simulink library "DSCdq_Library"  (R2018a)
settings: Solver=VariableStepAuto  StartTime=0.0  StopTime=10.0  RelTol=1e-3
values from neighbouring files (symbols this model uses):
  Ts = Ts_control / 60    (= 9.25925925926e-07)    [Equivalency_Script.m]    (also in FreqAdaptiveFFT_Script.m; FreqAdaptive_Script.m; ShortPulse_Script.m)
undefined symbols (not defined in the file or in its folder): ESS, PCC
libraries: $bdroot x20, powerlib_meascontrol x16, powerlib x3, cstblocks x2
settings Model: Creator=daniemot  LastModifiedBy=daniemot

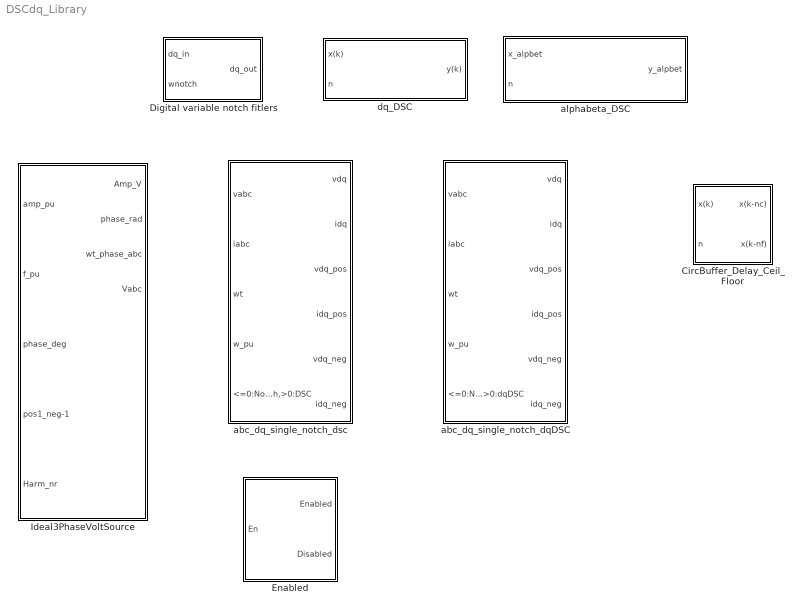
== system DSCdq_Library ==
  CircBuffer_Delay_Ceil_Floor : Subsystem  TreatAsAtomicUnit=on  SystemSampleTime=Ts  mask(Circular buffer with two variable delays (ceiling and floor)){Ts=Ts, nmax=200}
      mask prompts: Ts "Sampling time [s]"; nmax "Circular buffer length"
      mask help:
      | Circular Buffer
      | By: Mota
      | Revision history:	2021-07-16: first release
      |
      | Interface
      | Inputs
      | 	x : must be a vector pf two values
      | 	n : delay in samples (float, ideal delay is time was continuous)
      | 	nmax : max size of circular buffer, ONLY used in FIRST CYCLE
      |
      | Output
      | 	yc = x(k - ceil(n))
      | 	yf = x(k - floor(n))
  Digital variable notch fitlers : Subsystem  mask{Ts=Ts, zeta=0.707}
      mask prompts: Ts "Sampling time [s]"; zeta "Damping factor zeta for notches"
  Enabled : Subsystem  SystemSampleTime=Ts  mask(Enabled block){}
      mask help:
      | if En > 0
      |     Enabled = 1;
      |     Disabled = 0;
      | else
      |     Enabled = 0;
      |     Disabled = 1;
      | end
      mask Display: fprintf('Enable');
  Ideal3PhaseVoltSource : Subsystem  mask(Three-phase ideal voltage source){BaseAmp=1, fn=50}
      mask prompts: BaseAmp "Base phase-to-neutral amplitude [V]"; fn "Base frequency [Hz]"
      mask help:
      | Three-phase balanced ideal voltage source with neutral point not connected.
      |
      | The voltage source can be connected in series with others.
      |
      | va [V] = amp_pu*BaseAmp*sin(2*pi*(f_pu/s)*Harm_nr + Harm_nr*phase_deg*pi/180)
      | vb [V] = ... + Harm_nr*Ph_b_sign*2*pi/3)
      | vc [V] = ... + Harm_nr*Ph_c_sign*2*pi/3)
      |
      | If Pos1_Neg-1 = 1
      | 	Ph_b_sign = -1
      | 	Ph_c_sign = +1
      |
      | If Pos1_Neg-1 = -1
      | 	Ph_b_sign = +1
      | 	Ph_c_sign = -1
  abc_dq_single_notch_dqDSC : Subsystem  mask(abc->dq with Matlab){Ts=0.001, fn=50, fmin=40, zeta=0.707}
      mask prompts: Ts "Sampling time [s]"; fn "Grid frequency [Hz]"; fmin "Min. acceptable grid freq. [Hz]"; zeta "Zeta for notch filters"
      mask help:
      | To be done
      |
      | Max buffer size for DSC 500 samples
  abc_dq_single_notch_dsc : Subsystem  mask(abc->dq with Matlab){Ts=0.001, fn=50, fmin=40, zeta=0.707}
      mask prompts: Ts "Sampling time [s]"; fn "Rated grid frequency [Hz]"; fmin "Min. acceptable grid freq. [Hz]"; zeta "Zeta for notch filters"
      mask help:
      | To be done
      |
      | Max buffer size for DSC 500 samples
  alphabeta_DSC : Subsystem  mask{Ts=Ts, nmax=200}
      mask prompts: Ts "Sample times [s]"; nmax "Maximum delay nmax:"
      mask Display: fprintf('y(k)=0.5(x(k)+jx(k-n))');
  dq_DSC : Subsystem  mask{Ts=Ts, nmax=200}
      mask prompts: Ts "Sample times [s]"; nmax "Maximum delay nmax:"
      mask Display: fprintf('y(k)=0.5(x(k)+x(k-n))');

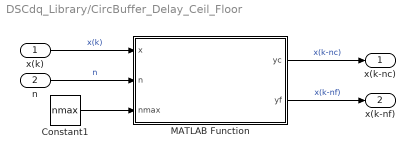
== system DSCdq_Library/CircBuffer_Delay_Ceil_Floor ==
  x(k) : Inport
  n : Inport  Port=2
  Constant1 : Constant  Value=nmax
  MATLAB Function : MATLAB Function  TreatAsAtomicUnit=on  SystemSampleTime=Ts
  x(k-nc) : Outport
  x(k-nf) : Outport  Port=2
  wires:
  n/1 -> MATLAB Function/2(n)  "n"
  MATLAB Function/2(yf) -> x(k-nf)/1  "x(k-nf)"
  x(k)/1 -> MATLAB Function/1(x)  "x(k)"
  MATLAB Function/1(yc) -> x(k-nc)/1  "x(k-nc)"
  Constant1/1 -> MATLAB Function/3(nmax)

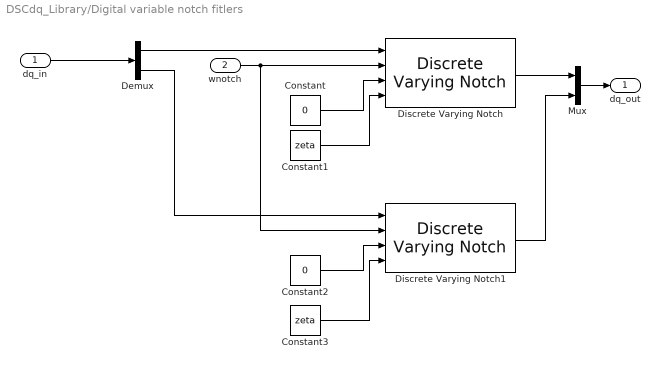
== system DSCdq_Library/Digital variable notch fitlers ==
  dq_in : Inport
  wnotch : Inport  Port=2
  Constant : Constant  Value=0
  Constant1 : Constant  Value=zeta
  Constant2 : Constant  Value=0
  Constant3 : Constant  Value=zeta
  Demux : Demux  Outputs=2
  Discrete Varying Notch : cstblocks/Linear Parameter Varying/Discrete Varying Notch  w0=0  Ts=Ts
      settings: SourceProductName=Control System Toolbox  SourceProductBaseCode=CT
  Discrete Varying Notch1 : cstblocks/Linear Parameter Varying/Discrete Varying Notch  w0=0  Ts=Ts
      settings: SourceProductName=Control System Toolbox  SourceProductBaseCode=CT
  Mux : Mux  Inputs=2
  dq_out : Outport
  wires:
  Constant/1 -> Discrete Varying Notch/3
  Constant1/1 -> Discrete Varying Notch/4
  Demux/2 -> Discrete Varying Notch1/1
  dq_in/1 -> Demux/1
  Constant2/1 -> Discrete Varying Notch1/3
  wnotch/1 -> Discrete Varying Notch1/2, Discrete Varying Notch/2
  Constant3/1 -> Discrete Varying Notch1/4
  Demux/1 -> Discrete Varying Notch/1
  Discrete Varying Notch/1 -> Mux/1
  Mux/1 -> dq_out/1
  Discrete Varying Notch1/1 -> Mux/2

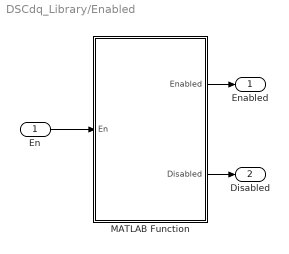
== system DSCdq_Library/Enabled ==
  En : Inport
  MATLAB Function : MATLAB Function  SystemSampleTime=Ts
      settings: RTWSystemCode=Inline
  Enabled : Outport
  Disabled : Outport  Port=2
  wires:
  En/1 -> MATLAB Function/1(En)
  MATLAB Function/1(Enabled) -> Enabled/1
  MATLAB Function/2(Disabled) -> Disabled/1

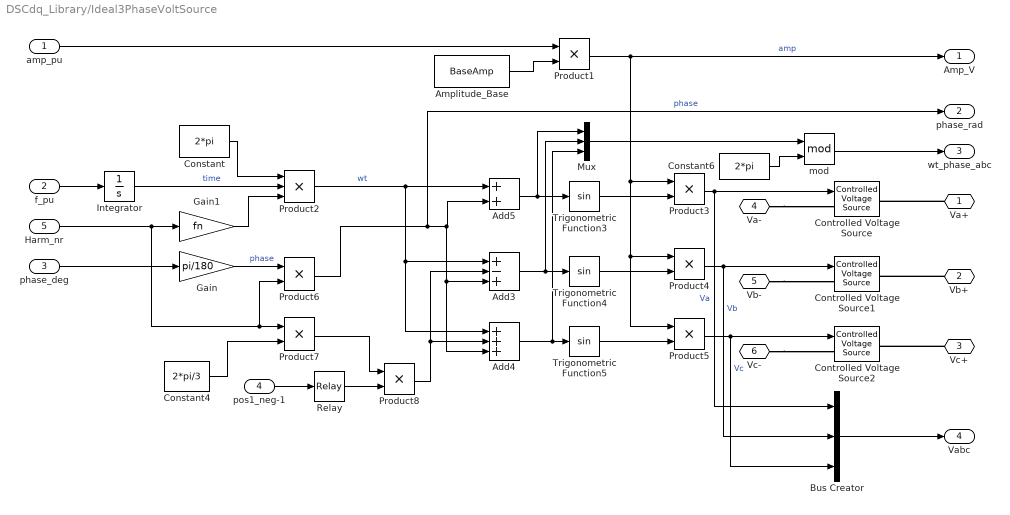
== system DSCdq_Library/Ideal3PhaseVoltSource ==
  amp_pu : Inport
  f_pu : Inport  Port=2
  phase_deg : Inport  Port=3
  pos1_neg-1 : Inport  Port=4
  Harm_nr : Inport  Port=5
  Add3 : Sum  Inputs=+-+
  Add4 : Sum  Inputs=+++
  Add5 : Sum
  Amplitude_Base : Constant  Value=BaseAmp
  Bus Creator : BusCreator  Inputs=3
  Constant : Constant  Value=2*pi
  Constant4 : Constant  Value=2*pi/3
  Constant6 : Constant  Value=2*pi
  Controlled Voltage Source : powerlib/Electrical Sources/Controlled Voltage Source  Initialize=off  Source_Type=AC  Amplitude=ESS.LSC.Ub*(2/3)^0.5  Phase=0  Frequency=PCC.fn  Measurements=None
  Controlled Voltage Source1 : powerlib/Electrical Sources/Controlled Voltage Source  Initialize=off  Source_Type=AC  Amplitude=ESS.LSC.Ub*(2/3)^0.5  Phase=-120  Frequency=PCC.fn  Measurements=None
  Controlled Voltage Source2 : powerlib/Electrical Sources/Controlled Voltage Source  Initialize=off  Source_Type=AC  Amplitude=ESS.LSC.Ub*(2/3)^0.5  Phase=120  Frequency=PCC.fn  Measurements=None
  Gain : Gain  Gain=pi/180
  Gain1 : Gain  Gain=fn
  Integrator : Integrator
  Mux : Mux  Inputs=3
  Product{1,3..8} (7 alike) : Product
  Product2 : Product  Inputs=3
  Relay : Relay  OnSwitchValue=0  OffSwitchValue=-0.1  OffOutputValue=-1
  Trigonometric Function3 : Trigonometry
  Trigonometric Function4 : Trigonometry
  Trigonometric Function5 : Trigonometry
  mod : Math  Operator=mod  SaturateOnIntegerOverflow=on
  Va+ : PMIOPort  Side=Right
  Vb+ : PMIOPort  Port=2  Side=Right
  Vc+ : PMIOPort  Port=3  Side=Right
  Va- : PMIOPort  Port=4  Side=Right
  Vb- : PMIOPort  Port=5  Side=Right
  Vc- : PMIOPort  Port=6  Side=Right
  Amp_V : Outport
  phase_rad : Outport  Port=2
  wt_phase_abc : Outport  Port=3
  Vabc : Outport  Port=4
  wires:
  Add4/1 -> Mux/3, Trigonometric Function5/1
  Product6/1 -> phase_rad/1, Add4/3, Add3/3, Add5/2  "phase"
  Add3/1 -> Mux/2, Trigonometric Function4/1
  pos1_neg-1/1 -> Relay/1
  Product3/1 -> Bus Creator/1, Controlled Voltage Source/1  "Va"
  amp_pu/1 -> Product1/1
  Product8/1 -> Add3/2, Add4/2
  Product5/1 -> Bus Creator/3, Controlled Voltage Source2/1  "Vc"
  Product4/1 -> Bus Creator/2, Controlled Voltage Source1/1  "Vb"
  Amplitude_Base/1 -> Product1/2
  Product7/1 -> Product8/1
  Product1/1 -> Product5/1, Product4/1, Product3/1, Amp_V/1  "amp"
  Relay/1 -> Product8/2
  Trigonometric Function3/1 -> Product3/2
  Product2/1 -> Add5/1, Add4/1, Add3/1  "wt"
  Trigonometric Function5/1 -> Product5/2
  Add5/1 -> Mux/1, Trigonometric Function3/1
  Trigonometric Function4/1 -> Product4/2
  phase_deg/1 -> Gain/1
  f_pu/1 -> Integrator/1
  Constant/1 -> Product2/1
  Gain1/1 -> Product2/3
  Bus Creator/1 -> Vabc/1
  Constant6/1 -> mod/2
  mod/1 -> wt_phase_abc/1
  Gain/1 -> Product6/1  "phase"
  Constant4/1 -> Product7/2
  Mux/1 -> mod/1
  Harm_nr/1 -> Product7/1, Product6/2, Gain1/1
  Integrator/1 -> Product2/2  "time"
  connections:
  Vb+/RConn1 -- Controlled Voltage Source1/RConn1
  Vc+/RConn1 -- Controlled Voltage Source2/RConn1
  Va+/RConn1 -- Controlled Voltage Source/RConn1
  Va-/RConn1 -- Controlled Voltage Source/LConn1
  Vb-/RConn1 -- Controlled Voltage Source1/LConn1
  Vc-/RConn1 -- Controlled Voltage Source2/LConn1

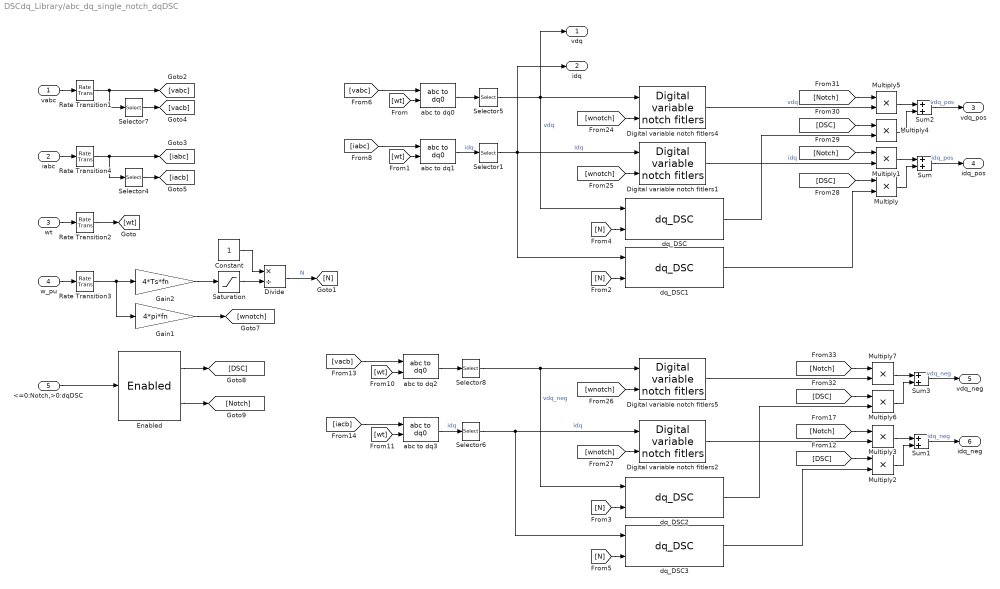
== system DSCdq_Library/abc_dq_single_notch_dqDSC ==
  vabc : Inport
  iabc : Inport  Port=2
  wt : Inport  Port=3
  w_pu : Inport  Port=4
  <=0:Notch,>0:dqDSC : Inport  Port=5
  Constant : Constant
  Digital variable notch fitlers{1..2,4..5} (4 alike) : $bdroot/Digital variable notch fitlers  Ts=Ts  zeta=zeta
  Divide : Product  Inputs=*/
  Enabled : $bdroot/Enabled
  Gain1 : Gain  Gain=4*pi*fn
  Gain2 : Gain  Gain=4*Ts*fn
  Multiply{,1..7} (8 alike) : Product
  Rate Transition1 : RateTransition  OutPortSampleTime=Ts
  Rate Transition2 : RateTransition  OutPortSampleTime=Ts
  Rate Transition3 : RateTransition  InitialCondition=1  OutPortSampleTime=Ts
  Rate Transition4 : RateTransition  OutPortSampleTime=Ts
  Saturation : Saturate  UpperLimit=inf  LowerLimit=0.000001
  Selector{1,5..6,8} (4 alike) : Selector  InputPortWidth=3  IndexOptions=Index vector (dialog)  Indices=[1 2]  OutputSizes=1
  Selector4 : Selector  InputPortWidth=3  IndexOptions=Index vector (dialog)  Indices=[1 3 2]  OutputSizes=1
  Selector7 : Selector  InputPortWidth=3  IndexOptions=Index vector (dialog)  Indices=[1 3 2]  OutputSizes=1
  Sum{,1..3} (4 alike) : Sum
  abc to dq{0..3} (4 alike) : powerlib_meascontrol/Transformations/abc to dq0  Alignment=90 degrees behind phase A axis
  dq_DSC{,1..3} (4 alike) : $bdroot/dq_DSC  Ts=Ts  nmax=round(1/(4*fmin*Ts))
  vdq : Outport
  idq : Outport  Port=2
  vdq_pos : Outport  Port=3
  idq_pos : Outport  Port=4
  vdq_neg : Outport  Port=5
  idq_neg : Outport  Port=6
  wires:
  wt/1 -> Rate Transition2/1
  abc to dq1/1 -> Selector1/1  "idq"
  Selector5/1 -> Digital variable notch fitlers4/1, vdq/1, dq_DSC/1  "vdq"
  abc to dq0/1 -> Selector5/1
  Selector1/1 -> Digital variable notch fitlers1/1, idq/1, dq_DSC1/1  "idq"
  [vabc] -> abc to dq0/1
  [iabc] -> abc to dq1/1
  vabc/1 -> Rate Transition1/1
  iabc/1 -> Rate Transition4/1
  Digital variable notch fitlers4/1 -> Multiply5/2  "vdq"
  Digital variable notch fitlers1/1 -> Multiply1/2  "idq"
  Sum2/1 -> vdq_pos/1  "vdq_pos"
  Sum/1 -> idq_pos/1  "idq_pos"
  Rate Transition2/1 -> [wt]
  [wt] -> abc to dq0/2
  [wt] -> abc to dq1/2
  Divide/1 -> [N]  "N"
  Rate Transition1/1 -> Selector7/1, [vabc]
  Selector7/1 -> [vacb]
  Rate Transition4/1 -> Selector4/1, [iabc]
  Selector4/1 -> [iacb]
  [wt] -> abc to dq3/2
  abc to dq2/1 -> Selector8/1
  Selector8/1 -> Digital variable notch fitlers5/1, dq_DSC2/1  "vdq_neg"
  [vacb] -> abc to dq2/1
  [wt] -> abc to dq2/2
  abc to dq3/1 -> Selector6/1  "idq"
  [iacb] -> abc to dq3/1
  Sum3/1 -> vdq_neg/1  "vdq_neg"
  Sum1/1 -> idq_neg/1  "idq_neg"
  Digital variable notch fitlers5/1 -> Multiply7/2
  Selector6/1 -> Digital variable notch fitlers2/1, dq_DSC3/1  "idq"
  Digital variable notch fitlers2/1 -> Multiply3/2
  dq_DSC3/1 -> Multiply2/2
  Gain2/1 -> Saturation/1
  Saturation/1 -> Divide/2
  Constant/1 -> Divide/1
  Rate Transition3/1 -> Gain1/1, Gain2/1
  w_pu/1 -> Rate Transition3/1
  Gain1/1 -> [wnotch]
  [wnotch] -> Digital variable notch fitlers4/2
  [wnotch] -> Digital variable notch fitlers1/2
  [wnotch] -> Digital variable notch fitlers5/2
  [wnotch] -> Digital variable notch fitlers2/2
  <=0:Notch,>0:dqDSC/1 -> Enabled/1
  Enabled/1 -> [DSC]
  Enabled/2 -> [Notch]
  [DSC] -> Multiply/1
  [Notch] -> Multiply1/1
  Multiply1/1 -> Sum/1
  Multiply/1 -> Sum/2
  [Notch] -> Multiply3/1
  [DSC] -> Multiply2/1
  Multiply3/1 -> Sum1/1
  Multiply2/1 -> Sum1/2
  [Notch] -> Multiply5/1
  Multiply4/1 -> Sum2/2
  [DSC] -> Multiply4/1
  Multiply5/1 -> Sum2/1
  [Notch] -> Multiply7/1
  Multiply6/1 -> Sum3/2
  [DSC] -> Multiply6/1
  Multiply7/1 -> Sum3/1
  [N] -> dq_DSC/2
  [N] -> dq_DSC1/2
  dq_DSC1/1 -> Multiply/2
  [N] -> dq_DSC3/2
  dq_DSC/1 -> Multiply4/2
  [N] -> dq_DSC2/2
  dq_DSC2/1 -> Multiply6/2

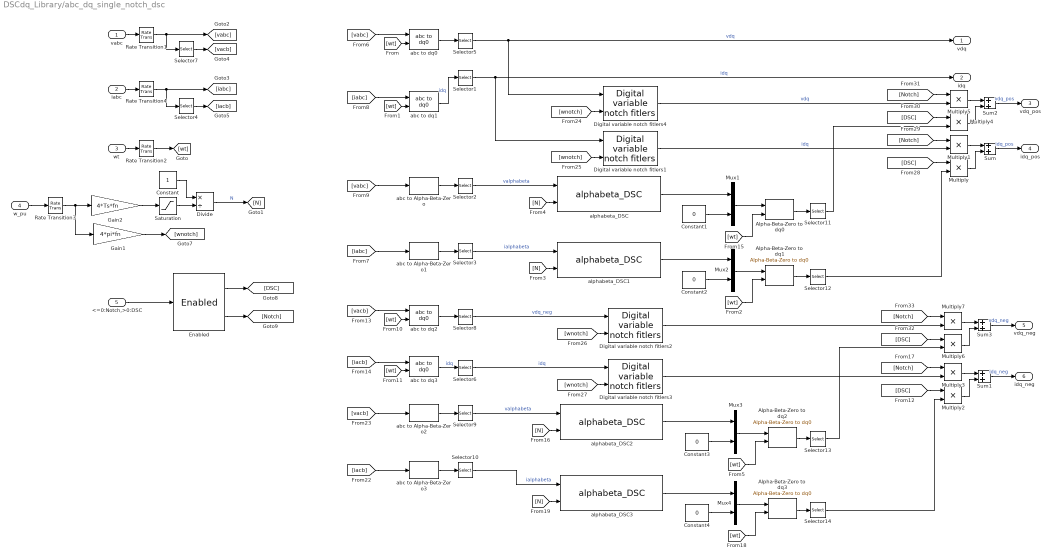
== system DSCdq_Library/abc_dq_single_notch_dsc ==
  vabc : Inport
  iabc : Inport  Port=2
  wt : Inport  Port=3
  w_pu : Inport  Port=4
  <=0:Notch,>0:DSC : Inport  Port=5
  Alpha-Beta-Zero to dq{0..3} (4 alike) : powerlib_meascontrol/Transformations/Alpha-Beta-Zero to dq0  Alignment=90 degrees behind phase A axis
      settings: SourceProductName=Simscape Power Systems
  Constant : Constant
  Constant{1..4} (4 alike) : Constant  Value=0
  Digital variable notch fitlers{1..4} (4 alike) : $bdroot/Digital variable notch fitlers  Ts=Ts  zeta=zeta
  Divide : Product  Inputs=*/
  Enabled : $bdroot/Enabled
  Gain1 : Gain  Gain=4*pi*fn
  Gain2 : Gain  Gain=4*Ts*fn
  Multiply{,1..7} (8 alike) : Product
  Mux{1..4} (4 alike) : Mux  Inputs=[2 1]
  Rate Transition1 : RateTransition  OutPortSampleTime=Ts
  Rate Transition2 : RateTransition  OutPortSampleTime=Ts
  Rate Transition3 : RateTransition  InitialCondition=1  OutPortSampleTime=Ts
  Rate Transition4 : RateTransition  OutPortSampleTime=Ts
  Saturation : Saturate  UpperLimit=inf  LowerLimit=0.000001
  Selector{1..3,5..6,8..14} (12 alike) : Selector  InputPortWidth=3  IndexOptions=Index vector (dialog)  Indices=[1 2]  OutputSizes=1
  Selector4 : Selector  InputPortWidth=3  IndexOptions=Index vector (dialog)  Indices=[1 3 2]  OutputSizes=1
  Selector7 : Selector  InputPortWidth=3  IndexOptions=Index vector (dialog)  Indices=[1 3 2]  OutputSizes=1
  Sum{,1..3} (4 alike) : Sum
  abc to Alpha-Beta-Zero{,1..3} (4 alike) : powerlib_meascontrol/Transformations/abc to Alpha-Beta-Zero
      settings: SourceProductName=Simscape Power Systems
  abc to dq{0..3} (4 alike) : powerlib_meascontrol/Transformations/abc to dq0  Alignment=90 degrees behind phase A axis
  alphabeta_DSC{,1..3} (4 alike) : $bdroot/alphabeta_DSC  Ts=Ts  nmax=round(1/(4*fmin*Ts))
  vdq : Outport
  idq : Outport  Port=2
  vdq_pos : Outport  Port=3
  idq_pos : Outport  Port=4
  vdq_neg : Outport  Port=5
  idq_neg : Outport  Port=6
  wires:
  wt/1 -> Rate Transition2/1
  abc to dq1/1 -> Selector1/1  "idq"
  Selector5/1 -> Digital variable notch fitlers4/1, vdq/1  "vdq"
  abc to dq0/1 -> Selector5/1
  Selector1/1 -> Digital variable notch fitlers1/1, idq/1  "idq"
  abc to Alpha-Beta-Zero/1 -> Selector2/1
  abc to Alpha-Beta-Zero1/1 -> Selector3/1
  Selector11/1 -> Multiply4/2
  Selector3/1 -> alphabeta_DSC1/1  "ialphabeta"
  [vabc] -> abc to dq0/1
  [iabc] -> abc to dq1/1
  vabc/1 -> Rate Transition1/1
  iabc/1 -> Rate Transition4/1
  Selector2/1 -> alphabeta_DSC/1  "valphabeta"
  Digital variable notch fitlers4/1 -> Multiply5/2  "vdq"
  Digital variable notch fitlers1/1 -> Multiply1/2  "idq"
  Selector12/1 -> Multiply/2
  Sum2/1 -> vdq_pos/1  "vdq_pos"
  Sum/1 -> idq_pos/1  "idq_pos"
  Rate Transition2/1 -> [wt]
  [wt] -> abc to dq0/2
  [wt] -> abc to dq1/2
  Divide/1 -> [N]  "N"
  Rate Transition1/1 -> Selector7/1, [vabc]
  Selector7/1 -> [vacb]
  Rate Transition4/1 -> Selector4/1, [iabc]
  Selector4/1 -> [iacb]
  [vabc] -> abc to Alpha-Beta-Zero/1
  [iabc] -> abc to Alpha-Beta-Zero1/1
  [wt] -> abc to dq3/2
  abc to dq2/1 -> Selector8/1
  Selector8/1 -> Digital variable notch fitlers2/1  "vdq_neg"
  [vacb] -> abc to dq2/1
  [wt] -> abc to dq2/2
  abc to dq3/1 -> Selector6/1  "idq"
  [iacb] -> abc to dq3/1
  Sum3/1 -> vdq_neg/1  "vdq_neg"
  Sum1/1 -> idq_neg/1  "idq_neg"
  Digital variable notch fitlers2/1 -> Multiply7/2
  Selector6/1 -> Digital variable notch fitlers3/1  "idq"
  Digital variable notch fitlers3/1 -> Multiply3/2
  abc to Alpha-Beta-Zero3/1 -> Selector10/1
  Selector10/1 -> alphabeta_DSC3/1  "ialphabeta"
  abc to Alpha-Beta-Zero2/1 -> Selector9/1
  [iacb] -> abc to Alpha-Beta-Zero3/1
  [vacb] -> abc to Alpha-Beta-Zero2/1
  Alpha-Beta-Zero to dq2/1 -> Selector13/1
  Selector9/1 -> alphabeta_DSC2/1  "valphabeta"
  Alpha-Beta-Zero to dq3/1 -> Selector14/1
  Gain2/1 -> Saturation/1
  Saturation/1 -> Divide/2
  Constant/1 -> Divide/1
  Rate Transition3/1 -> Gain1/1, Gain2/1
  w_pu/1 -> Rate Transition3/1
  Gain1/1 -> [wnotch]
  [wnotch] -> Digital variable notch fitlers4/2
  [wnotch] -> Digital variable notch fitlers1/2
  [wnotch] -> Digital variable notch fitlers2/2
  [wnotch] -> Digital variable notch fitlers3/2
  <=0:Notch,>0:DSC/1 -> Enabled/1
  Enabled/1 -> [DSC]
  Enabled/2 -> [Notch]
  [DSC] -> Multiply/1
  [Notch] -> Multiply1/1
  Multiply1/1 -> Sum/1
  Multiply/1 -> Sum/2
  [Notch] -> Multiply3/1
  [DSC] -> Multiply2/1
  Multiply3/1 -> Sum1/1
  Multiply2/1 -> Sum1/2
  [Notch] -> Multiply5/1
  Multiply4/1 -> Sum2/2
  [DSC] -> Multiply4/1
  Multiply5/1 -> Sum2/1
  [Notch] -> Multiply7/1
  Multiply6/1 -> Sum3/2
  [DSC] -> Multiply6/1
  Multiply7/1 -> Sum3/1
  Mux1/1 -> Alpha-Beta-Zero to dq0/1
  Alpha-Beta-Zero to dq0/1 -> Selector11/1
  [wt] -> Alpha-Beta-Zero to dq0/2
  Constant1/1 -> Mux1/2
  alphabeta_DSC/1 -> Mux1/1
  [N] -> alphabeta_DSC/2
  [wt] -> Alpha-Beta-Zero to dq1/2
  Alpha-Beta-Zero to dq1/1 -> Selector12/1
  Mux2/1 -> Alpha-Beta-Zero to dq1/1
  alphabeta_DSC1/1 -> Mux2/1
  Constant2/1 -> Mux2/2
  [N] -> alphabeta_DSC1/2
  Mux3/1 -> Alpha-Beta-Zero to dq2/1
  Constant3/1 -> Mux3/2
  [wt] -> Alpha-Beta-Zero to dq2/2
  [N] -> alphabeta_DSC2/2
  alphabeta_DSC2/1 -> Mux3/1
  Mux4/1 -> Alpha-Beta-Zero to dq3/1
  Constant4/1 -> Mux4/2
  [wt] -> Alpha-Beta-Zero to dq3/2
  [N] -> alphabeta_DSC3/2
  alphabeta_DSC3/1 -> Mux4/1
  Selector13/1 -> Multiply6/2
  Selector14/1 -> Multiply2/2

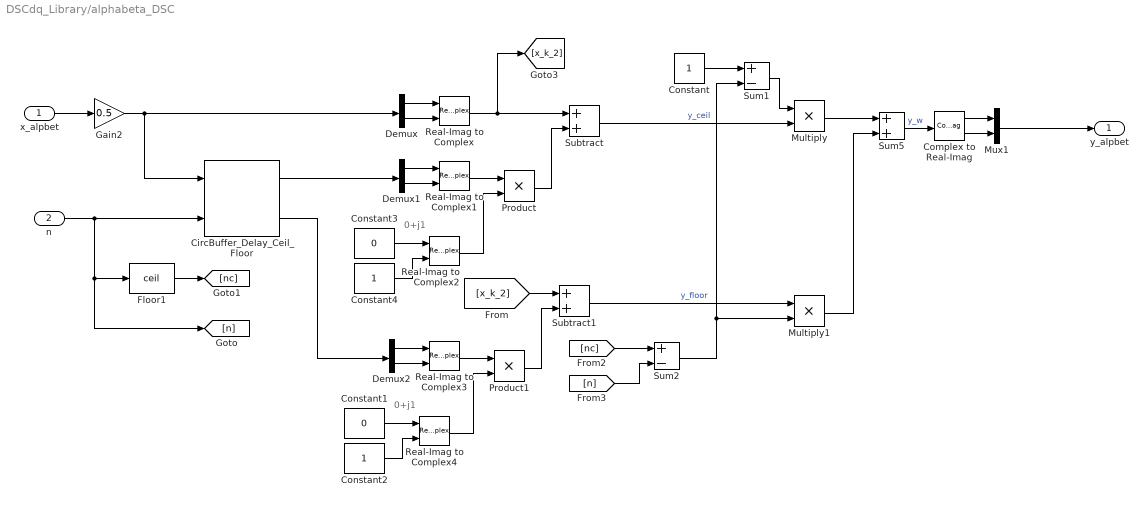
== system DSCdq_Library/alphabeta_DSC ==
  note: 0+j1
  note: 0+j1
  x_alpbet : Inport
  n : Inport  Port=2
  CircBuffer_Delay_Ceil_Floor : $bdroot/CircBuffer_Delay_Ceil_Floor  Ts=Ts  nmax=200
  Complex to Real-Imag : ComplexToRealImag
  Constant : Constant
  Constant1 : Constant  Value=0
  Constant2 : Constant
  Constant3 : Constant  Value=0
  Constant4 : Constant
  Demux : Demux  Outputs=2
  Demux1 : Demux  Outputs=2
  Demux2 : Demux  Outputs=2
  Floor1 : Rounding  Operator=ceil
  Gain2 : Gain  Gain=0.5
  Multiply : Product
  Multiply1 : Product
  Mux1 : Mux  Inputs=[1 1]
  Product : Product
  Product1 : Product
  Real-Imag to Complex{,1..4} (5 alike) : RealImagToComplex
  Subtract : Sum
  Subtract1 : Sum
  Sum1 : Sum  Inputs=+-
  Sum2 : Sum  Inputs=+-
  Sum5 : Sum
  y_alpbet : Outport
  wires:
  Complex to Real-Imag/2 -> Mux1/2
  Mux1/1 -> y_alpbet/1
  Demux/1 -> Real-Imag to Complex/1
  Product/1 -> Subtract/2
  x_alpbet/1 -> Gain2/1
  Demux/2 -> Real-Imag to Complex/2
  CircBuffer_Delay_Ceil_Floor/1 -> Demux1/1
  Complex to Real-Imag/1 -> Mux1/1
  Demux1/2 -> Real-Imag to Complex1/2
  Constant4/1 -> Real-Imag to Complex2/2
  n/1 -> Floor1/1, [n], CircBuffer_Delay_Ceil_Floor/2
  Real-Imag to Complex/1 -> [x_k_2], Subtract/1
  Constant3/1 -> Real-Imag to Complex2/1
  Real-Imag to Complex1/1 -> Product/1
  Demux1/1 -> Real-Imag to Complex1/1
  Real-Imag to Complex2/1 -> Product/2
  [nc] -> Sum2/1
  Sum2/1 -> Multiply1/2, Sum1/2
  Subtract1/1 -> Multiply1/1  "y_floor"
  Subtract/1 -> Multiply/2  "y_ceil"
  Multiply/1 -> Sum5/1
  Multiply1/1 -> Sum5/2
  Sum1/1 -> Multiply/1
  [n] -> Sum2/2
  Constant/1 -> Sum1/1
  Floor1/1 -> [nc]
  Demux2/1 -> Real-Imag to Complex3/1
  Constant1/1 -> Real-Imag to Complex4/1
  Demux2/2 -> Real-Imag to Complex3/2
  Constant2/1 -> Real-Imag to Complex4/2
  Product1/1 -> Subtract1/2
  Real-Imag to Complex3/1 -> Product1/1
  Real-Imag to Complex4/1 -> Product1/2
  CircBuffer_Delay_Ceil_Floor/2 -> Demux2/1
  Gain2/1 -> Demux/1, CircBuffer_Delay_Ceil_Floor/1
  [x_k_2] -> Subtract1/1
  Sum5/1 -> Complex to Real-Imag/1  "y_w"

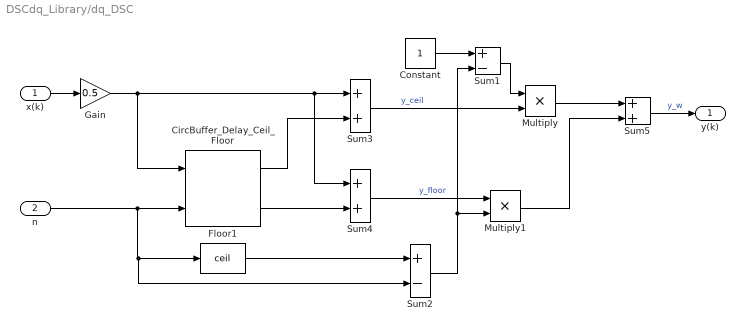
== system DSCdq_Library/dq_DSC ==
  x(k) : Inport
  n : Inport  Port=2
  CircBuffer_Delay_Ceil_Floor : $bdroot/CircBuffer_Delay_Ceil_Floor  Ts=Ts  nmax=nmax
  Constant : Constant
  Floor1 : Rounding  Operator=ceil
  Gain : Gain  Gain=0.5
  Multiply : Product
  Multiply1 : Product
  Sum1 : Sum  Inputs=+-
  Sum2 : Sum  Inputs=+-
  Sum3 : Sum
  Sum4 : Sum
  Sum5 : Sum
  y(k) : Outport
  wires:
  x(k)/1 -> Gain/1
  Sum3/1 -> Multiply/2  "y_ceil"
  Sum4/1 -> Multiply1/1  "y_floor"
  Constant/1 -> Sum1/1
  Sum2/1 -> Multiply1/2, Sum1/2
  Floor1/1 -> Sum2/1
  n/1 -> Sum2/2, Floor1/1, CircBuffer_Delay_Ceil_Floor/2
  Multiply1/1 -> Sum5/2
  Multiply/1 -> Sum5/1
  Sum1/1 -> Multiply/1
  Gain/1 -> Sum4/1, Sum3/1, CircBuffer_Delay_Ceil_Floor/1
  Sum5/1 -> y(k)/1  "y_w"
  CircBuffer_Delay_Ceil_Floor/1 -> Sum3/2
  CircBuffer_Delay_Ceil_Floor/2 -> Sum4/2

== matlab function DSCdq_Library/CircBuffer_Delay_Ceil_Floor/MATLAB Function ==
  data: x input; yc output; n input; yf output; nmax input
function [yc,    yf]  = CircBuff_Delay_CeilFloor(x, n, nmax)
%% %%%%%%%%%%%%%%%%%%%%%%%%%%%%%%%%%%%%%%%%%%%%%%%%%%%%%%%%%%%%%%%%%%%%%%%%
% Circular Buffer 
% By: Mota
% Revision history:
%       2021-07-16: first release
%
%%Interface  
%   Inputs
%       x : must be a vector pf two values
%       n : delay in samples (float, ideal delay is time was continuous)
%       nmax : max size of circular buffer, ONLY used in FIRST CYCLE
%
%   Output
%       yc = x(k - ceil(n))
%       yf = x(k - floor(n))
% 

persistent CB       % circular buffer, created with zeros in first cycle
persistent ins_p    % insertion pointer, integer, zero -> Nmax-1
persistent Nmax     % Buffer lenght, updated ONLY in FIRST CYCLE


%% Initialization of persistent variables
if isempty(Nmax)
    if nmax < 5     % Hardcoded minimum lenght of buffer (arbitrary)
        Nmax = 5;
    else 
        Nmax = round(nmax); % No limit for maximum lenght of buffer 
    end
    
    CB = zeros(Nmax, 2);    % circular buffer
                            % Nmax lines x 2 columns 
                            % Column 1: ceiling 
                            % Column 2: floor
    
    ins_p = 0;      % Insertion pointer initialization
    
end

%% %%%%%%%%%%%%%%%%%%%%%%%%%%%%%%%%%%%%%%%%%%%%%%%%%%%%%%%%%%%%%%%%%%%%%%
% Insertion of current values
%%%%%%%%%%%%%%%%%%%%%%%%%%%%%%%%%%%%%%%%%%%%%%%%%%%%%%%%%%%%%%%%%%%%%%%%%
CB(ins_p + 1, 1) = x(1);    
CB(ins_p + 1, 2) = x(2);

%% %%%%%%%%%%%%%%%%%%%%%%%%%%%%%%%%%%%%%%%%%%%%%%%%%%%%%%%%%%%%%%%%%%%%%%
% Retrieval pointer calculation
%   Be careful with confusion of indices
%       Matlab index for array:     1, 2,... Nmax
%       Insertion pointer values:   0, 1,... Nmax - 1
%%%%%%%%%%%%%%%%%%%%%%%%%%%%%%%%%%%%%%%%%%%%%%%%%%%%%%%%%%%%%%%%%%%%%%%%%
if n >= 1       
    if n <= Nmax - 1    % if 1 >= n >= Nmax - 1 
                        % n cannot be equal to Nmax, or else the retrieval
                        % pointers retreat back to the the insertion
                        % pointer.
                                
        p_r_c = mod(ins_p - ceil(n), Nmax); % ceiling retrieval pointer
        p_r_f = mod(ins_p - floor(n), Nmax); % floor retrieval pointer
    
    else
        % The maximum delay is Nmax - 1
        p_r_c = mod(ins_p - Nmax - 1, Nmax);
        p_r_f = mod(ins_p - Nmax - 1, Nmax);
    end
else
    % Minimul delay is zero
    p_r_c = ins_p;
    p_r_f = ins_p;
end
    
%% %%%%%%%%%%%%%%%%%%%%%%%%%%%%%%%%%%%%%%%%%%%%%%%%%%%%%%%%%%%%%%%%%%%%%%
% Temporary variables with retrieved values
%   CB indexes: 1, 2, ... Nmax
%%%%%%%%%%%%%%%%%%%%%%%%%%%%%%%%%%%%%%%%%%%%%%%%%%%%%%%%%%%%%%%%%%%%%%%%%
col1_c = CB(p_r_c + 1, 1); 
col1_f = CB(p_r_f + 1, 1);

col2_c = CB(p_r_c + 1, 2);
col2_f = CB(p_r_f + 1, 2);

%% %%%%%%%%%%%%%%%%%%%%%%%%%%%%%%%%%%%%%%%%%%%%%%%%%%%%%%%%%%%%%%%%%%%%%%
% Outputs vectors
%%%%%%%%%%%%%%%%%%%%%%%%%%%%%%%%%%%%%%%%%%%%%%%%%%%%%%%%%%%%%%%%%%%%%%%%%
yc = [col1_c col2_c];
yf = [col1_f col2_f];

%% %%%%%%%%%%%%%%%%%%%%%%%%%%%%%%%%%%%%%%%%%%%%%%%%%%%%%%%%%%%%%%%%%%%%%%
% Update Outputs vectors
%%%%%%%%%%%%%%%%%%%%%%%%%%%%%%%%%%%%%%%%%%%%%%%%%%%%%%%%%%%%%%%%%%%%%%%%%
ins_p = mod(ins_p + 1, Nmax);

== matlab function DSCdq_Library/Enabled/MATLAB Function ==
  data: En input; Enabled output; Disabled output
%%%%%%%%%%%%%%%%%%%%%%%%%%%%%%%%%%%%%%%%%%%%%%%%%%%%%%%%%%%%%%%%%%%%%%%%%%
% Enabled block
%%%%%%%%%%%%%%%%%%%%%%%%%%%%%%%%%%%%%%%%%%%%%%%%%%%%%%%%%%%%%%%%%%%%%%%%%%\

% Inputs
%   Enabled: if >0 enabled
% Output
%   Enabled: 1 if enabled, 0 if disabled
%   Disabled: 1 if disabled, 0 if enabled

%%%%%%%%%%%%%%%%%%%%%%%%%%%%%%%%%%%%%%%%%%%%%%%%%%%%%%%%%%%%%%%%%%%%%%%%%%\
% Prog/rev history
%   Mota - 2021-06-02: first release

function [Enabled,Disabled] = Enabled(En)

if En > 0
    Enabled = 1;
    Disabled = 0;
else
    Enabled = 0;
    Disabled = 1;
end
